simulink model "PD_I_Continuous"  (R2018a)
settings: Solver=ode4  StartTime=0.0  StopTime=30  FixedStep=0.02  RelTol=1e-3
libraries: fuzblock x1
settings Model: Creator=dell  LastModifiedBy=dell

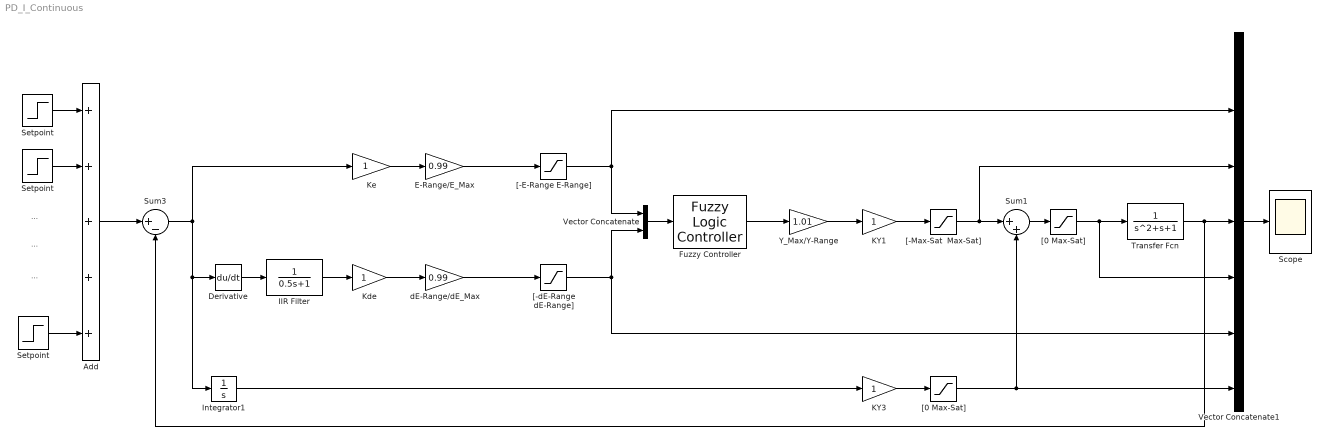
== system PD_I_Continuous ==
  note: ...
  note: ...
  note: ...
  "    Transfer Fcn   " : TransferFcn  Denominator=[1 1 1]
  Add : Sum  Inputs=+++++
  Derivative : Derivative
  E-Range/E_Max : Gain  Gain=0.99
  Fuzzy Controller : fuzblock/Fuzzy Logic  Controller  FIS='bgbg.fis'  OutputSampleNumber=1000  DataType=double  FuzzifiedInputs=off  RuleFiringStrengths=off  RuleOutputs=off  AggregatedOutputs=off  SimulateUsing=Interpreted execution  OutOfRangeInputValueMessage=warning  NoRuleFiredMessage=warning  EmptyOutputFuzzySetMessage=warning
  IIR Filter : TransferFcn  Denominator=[0.5 1]
  Integrator1 : Integrator
  "KY1 " : Gain
  KY3 : Gain
  "Kde " : Gain
  "Ke " : Gain
  "Scope " : Scope
  "Setpoint " : Step  Time=0  After=0  SampleTime=0.02
  "Setpoint " : Step  Time=0  After=50  SampleTime=0.02
  "Setpoint " : Step  Time=0  After=0  SampleTime=0.02
  Sum1 : Sum  Inputs=|++
  Sum3 : Sum  Inputs=|+-
  Vector Concatenate : Concatenate
  Vector Concatenate1 : Concatenate  NumInputs=7
  "Y_Max/Y-Range " : Gain  Gain=1.01
  "[-E-Range E-Range] " : Saturate  UpperLimit=99  LowerLimit=-99  LinearizeAsGain=off  OutMin=[-100]  OutMax=[100]
  "[-Max-Sat  Max-Sat] " : Saturate  UpperLimit=100  LowerLimit=-100  LinearizeAsGain=off
  "[-dE-Range dE-Range] " : Saturate  UpperLimit=99  LowerLimit=-99  LinearizeAsGain=off
  "[0 Max-Sat] " : Saturate  UpperLimit=100  LowerLimit=0  LinearizeAsGain=off
  "[0 Max-Sat] " : Saturate  UpperLimit=100  LowerLimit=0  LinearizeAsGain=off
  "dE-Range/dE_Max " : Gain  Gain=0.99
  wires:
  Vector Concatenate1/1 -> "Scope "/1
  E-Range/E_Max/1 -> "[-E-Range E-Range] "/1
  "Setpoint "/1 -> Add/5
  "[-E-Range E-Range] "/1 -> Vector Concatenate1/2, Vector Concatenate/1
  "Ke "/1 -> E-Range/E_Max/1
  "    Transfer Fcn   "/1 -> Vector Concatenate1/4, Sum3/2
  "dE-Range/dE_Max "/1 -> "[-dE-Range dE-Range] "/1
  "Y_Max/Y-Range "/1 -> "KY1 "/1
  Vector Concatenate/1 -> Fuzzy Controller/1
  Derivative/1 -> IIR Filter/1
  Integrator1/1 -> KY3/1
  Sum3/1 -> Integrator1/1, Derivative/1, "Ke "/1
  "Kde "/1 -> "dE-Range/dE_Max "/1
  Add/1 -> Sum3/1
  "[0 Max-Sat] "/1 -> Vector Concatenate1/5, "    Transfer Fcn   "/1
  Fuzzy Controller/1 -> "Y_Max/Y-Range "/1
  "Setpoint "/1 -> Add/2
  "Setpoint "/1 -> Add/1
  "KY1 "/1 -> "[-Max-Sat  Max-Sat] "/1
  KY3/1 -> "[0 Max-Sat] "/1
  Sum1/1 -> "[0 Max-Sat] "/1
  "[-dE-Range dE-Range] "/1 -> Vector Concatenate1/6, Vector Concatenate/2
  "[-Max-Sat  Max-Sat] "/1 -> Vector Concatenate1/3, Sum1/1
  "[0 Max-Sat] "/1 -> Vector Concatenate1/7, Sum1/2
  IIR Filter/1 -> "Kde "/1
